simulink model "bloco1"  (R2016a)
settings: Solver=VariableStepAuto  StartTime=0.0  StopTime=10.0  RelTol=1e-3
values from neighbouring files (symbols this model uses):
  b1 = 7    [Q1.m]
  b2 = 7    [Q1.m]
  F = 1    [Q1.m]
  k1 = 20    [Q1.m]
  k2 = 20    [Q1.m]
  m1 = 10    [Q1.m]
  m2 = 10    [Q1.m]
settings Model: Creator=diona  LastModifiedBy=diona

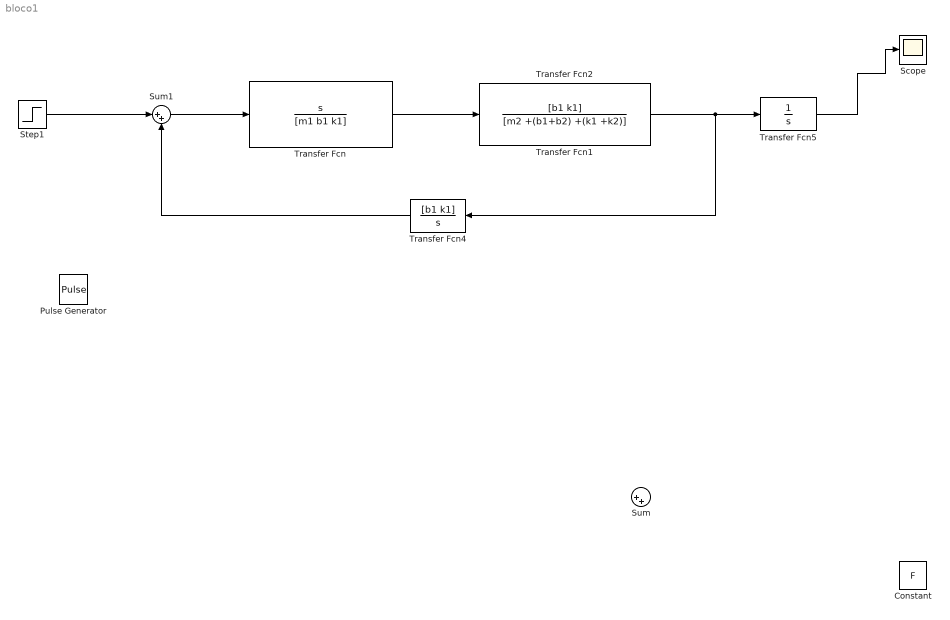
== system bloco1 ==
  Constant : Constant  Value=F
  Pulse Generator : DiscretePulseGenerator  PulseType=Time based  Period=10  PulseWidth=5
  Scope : Scope
  Step1 : Step  SampleTime=0
  Sum : Sum  Inputs=|++
  Sum1 : Sum  Inputs=|++
  Transfer Fcn : TransferFcn  Numerator=[1 0]  Denominator=[m1 b1 k1]
  Transfer Fcn1 : TransferFcn  Numerator=[b1 k1]  Denominator=[m2 +(b1+b2) +(k1 +k2)]
  Transfer Fcn2 : TransferFcn  Numerator=[b1 k1]  Denominator=[m2 +(b1+b2) +(k1 +k2)]
  Transfer Fcn4 : TransferFcn  Numerator=[b1 k1]  Denominator=[1 0]
  Transfer Fcn5 : TransferFcn  Denominator=[1 0]
  wires:
  Sum1/1 -> Transfer Fcn/1
  Transfer Fcn4/1 -> Sum1/2
  Transfer Fcn2/1 -> Transfer Fcn4/1, Transfer Fcn5/1
  Transfer Fcn/1 -> Transfer Fcn2/1
  Transfer Fcn5/1 -> Scope/1
  Step1/1 -> Sum1/1
